simulink model "coursework_v92"  (R2025a)
settings: Solver=VariableStepAuto  StartTime=0.0  StopTime=0.11  MaxStep=1e-5  RelTol=1e-6
undefined symbols (not defined in the file): dspblkCoreblockFVToolHelper, gcbh, k1, k2, ki, T
settings Model: Creator=zuimio  LastModifiedBy=zuimio

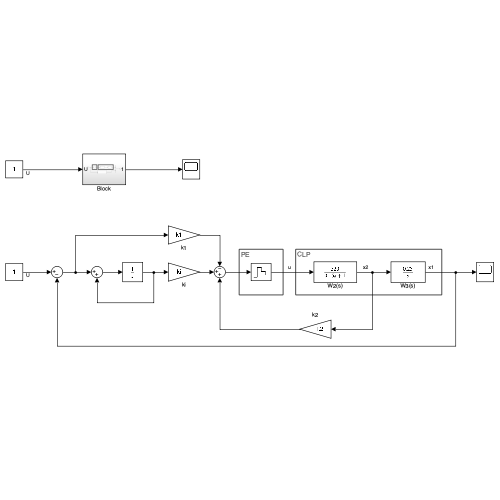
[thumbnail: Simulink's stored preview of the top-level diagram]
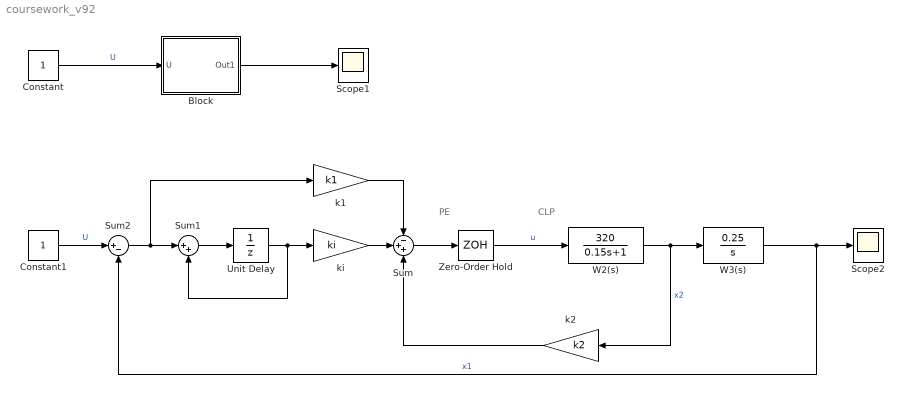
== system coursework_v92 ==
  note: CLP
  note: PE
  Block : Subsystem
  Constant : Constant
  Constant1 : Constant
  Scope1 : Scope
      settings: ActiveDisplayYMinimum=-1  ActiveDisplayYMaximum=1
  Scope2 : Scope
      settings: ActiveDisplayYMinimum=-0.16016312939352539  ActiveDisplayYMaximum=1.4414681645417289
  Sum : Sum  Inputs=-++
  Sum1 : Sum  Inputs=|++
  Sum2 : Sum  Inputs=|+-
  Unit Delay : UnitDelay  SampleTime=-1  HasFrameUpgradeWarning=on
  W2(s) : TransferFcn  Numerator=[320]  Denominator=[0.15 1]
  W3(s) : TransferFcn  Numerator=[0.25]  Denominator=[1 0]
  Zero-Order Hold : ZeroOrderHold  SampleTime=T
  k1 : Gain  Gain=k1
  k2 : Gain  Gain=k2
  ki : Gain  Gain=ki
  wires:
  Constant/1 -> Block/1(U)  "U"
  Block/1(Out1) -> Scope1/1
  W3(s)/1 -> Scope2/1, Sum2/2  "x1"
  Zero-Order Hold/1 -> W2(s)/1  "u"
  W2(s)/1 -> k2/1, W3(s)/1  "x2"
  k2/1 -> Sum/3
  Sum/1 -> Zero-Order Hold/1
  Sum2/1 -> k1/1, Sum1/1
  Sum1/1 -> Unit Delay/1
  Unit Delay/1 -> ki/1, Sum1/2
  ki/1 -> Sum/2
  k1/1 -> Sum/1
  Constant1/1 -> Sum2/1  "U"

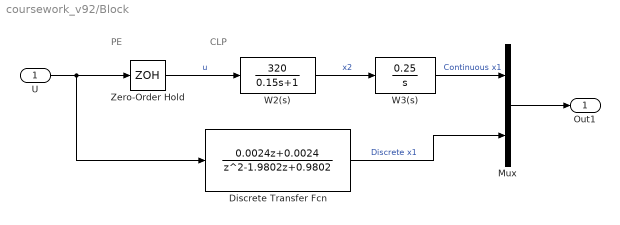
== system coursework_v92/Block ==
  note: CLP
  note: PE
  U : Inport
  Discrete Transfer Fcn : DiscreteTransferFcn  LoadFcn=dspblkCoreblockFVToolHelper(gcbh,'load');  Numerator=[0 0.0024 0.0024]  Denominator=[1 -1.9802 0.9802]
      settings: CopyFcn=dspblkCoreblockFVToolHelper(gcbh,'copy');  DeleteFcn=dspblkCoreblockFVToolHelper(gcbh,'close');  ModelCloseFcn=dspblkCoreblockFVToolHelper(gcbh,'close');  PreSaveFcn=dspblkCoreblockFVToolHelper(gcbh,'presave');  PostSaveFcn=dspblkCoreblockFVToolHelper(gcbh,'postsave');  CloseFcn=dspblkCoreblockFVToolHelper(gcbh,'close');
  Mux : Mux  Inputs=2
  W2(s) : TransferFcn  Numerator=[320]  Denominator=[0.15 1]
  W3(s) : TransferFcn  Numerator=[0.25]  Denominator=[1 0]
  Zero-Order Hold : ZeroOrderHold  SampleTime=T
  Out1 : Outport
  wires:
  W3(s)/1 -> Mux/1  "Continuous x1"
  Zero-Order Hold/1 -> W2(s)/1  "u"
  Discrete Transfer Fcn/1 -> Mux/2  "Discrete x1"
  U/1 -> Discrete Transfer Fcn/1, Zero-Order Hold/1
  Mux/1 -> Out1/1
  W2(s)/1 -> W3(s)/1  "x2"
